simulink model "SurroundVehicleSensorFusion"  (R2022b)
settings: Solver=FixedStepAuto  StartTime=0.0  StopTime=scenario.StopTime  RelTol=1e-3  EnableMultiTasking=on
undefined symbols (not defined in the file): M, N, P, Q, trackAssignmentThreshold
libraries: motalgorithmslib x1, trackingutilitieslib x1
settings Model: Creator=The MathWorks, Inc.  LastModifiedBy=joelmiranda
settings SolverCC: AlgebraicLoopSolver=TrustRegion  MaxZcPerStep=1
settings DataIOCC: SaveOutput=off  SaveTime=off  ReturnWorkspaceOutputs=off
settings OptimizationCC: DefaultParameterBehavior=Inlined  InlineInvariantSignals=on  EnhancedBackFolding=on  PassReuseOutputArgsAs=Individual arguments  ZeroExternalMemoryAtStartup=off  ZeroInternalMemoryAtStartup=off  EfficientFloat2IntCast=on  OptimizeBlockOrder=speed  DifferentSizesBufferReuse=on  OptimizationCustomize=off  EfficientTunableParamExpr=on
settings DebuggingCC: ParameterPrecisionLossMsg=none  ParameterTunabilityLossMsg=error  UnconnectedInputMsg=warning  UnconnectedOutputMsg=warning  UnconnectedLineMsg=warning  ModelReferenceSymbolNameMessage=none  PregeneratedLibrarySubsystemCodeDiagnostic=none  SFMachineParentedDataDiag=warning  ArithmeticOperatorsInVariantConditions=warning
settings HardwareCC: ProdLongLongMode=on
settings ModelReferenceCC: EnableRefExpFcnMdlSchedulingChecks=on  PropagateVarSize=During execution
settings SFSimCC: SimUseLocalCustomCode=off  SimTargetLang=C++
settings RTWCC: Description=Embedded Coder  SystemTargetFile=ert.tlc  TemplateMakefile=ert_default_tmf  RTWVerbose=off  RTWUseLocalCustomCode=off  BuildConfiguration=Faster Runs  CodeExecutionProfiling=on  CodeProfilingSaveOptions=AllData  TargetLang=C++  DLArmComputeVersion=19.05
settings CodeAppCC: ForceParamTrailComments=on  IgnoreCustomStorageClasses=off  OperatorAnnotations=on  SimulinkDataObjDesc=on  SFDataObjDesc=on  CustomSymbolStrGlobalVar=$N$M  CustomSymbolStrType=$N$M_T  CustomSymbolStrFcn=APV_$N$M$F  CustomSymbolStrMacro=$N$M  InsertBlockDesc=on
settings ERTTargetCC: TargetLangStandard=C++03 (ISO)  GenerateSampleERTMain=on  CombineSignalStateStructs=on  CodeInterfacePackaging=C++ class  SupportVariableSizeSignals=on  InlinedParameterPlacement=NonHierarchical  RootIOFormat=Structure reference  ERTCustomFileTemplate=example_file_process.tlc
settings ConfigComp: CovScope=ReferencedModels  CovIncludeTopModel=off

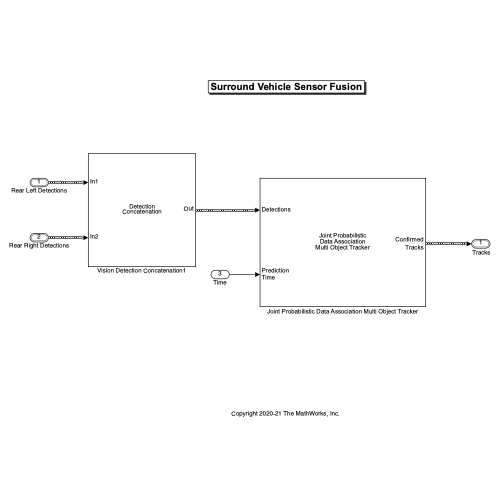
[thumbnail: Simulink's stored preview of the top-level diagram]
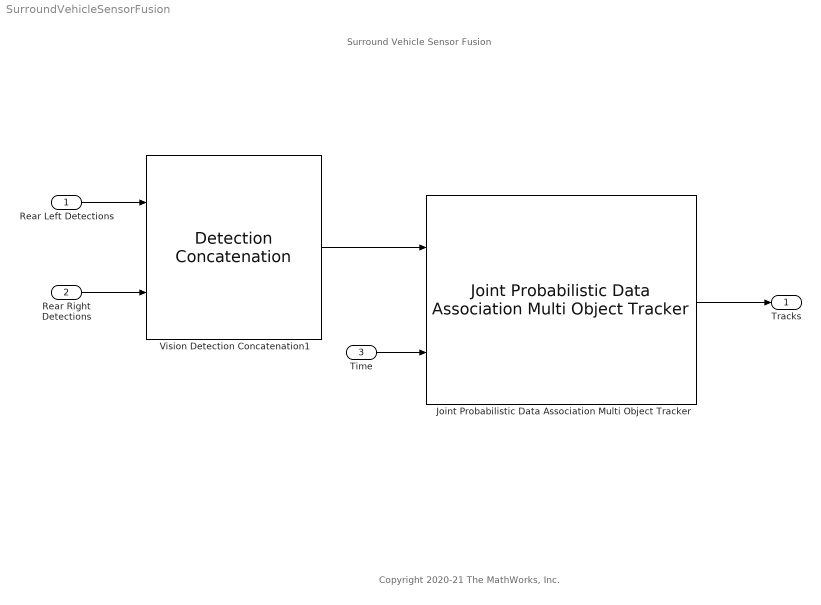
== system SurroundVehicleSensorFusion ==
  note: Surround Vehicle Sensor Fusion
  note: Copyright 2020-21 The MathWorks, Inc.
  Rear Left Detections : Inport  OutDataTypeStr=Bus: BusObjectDetections1  PortDimensions=[1 1]  SampleTime=[0.10000000000000001,0]  BusOutputAsStruct=on
  Rear Right Detections : Inport  Port=2  OutDataTypeStr=Bus: BusObjectDetections1  PortDimensions=[1 1]  SampleTime=[0.10000000000000001,0]  BusOutputAsStruct=on
  Time : Inport  Port=3  OutDataTypeStr=double  PortDimensions=[1 1]  SampleTime=[0.10000000000000001,0]
  Joint Probabilistic Data Association Multi Object Tracker : motalgorithmslib/Joint Probabilistic Data Association Multi Object Tracker  TrackerIndex=uint32( 0 )  FilterInitializationFcn=helperInitializeCVEKFFilter  MaxNumEvents=inf  EventGenerationFcn=jpdaEvents  MaxNumTracks=numTracks  MaxNumSensors=numSensors  TimeTolerance=1e-5  OOSMHandling=Terminate  MaxNumOOSMSteps=3  StateParametersSimulink=struct  HasStateParametersInput=off  EnableMemoryManagement=off  SimulateUsing=Interpreted execution  AssignmentThreshold=[ 1, Inf ] * trackAssignmentThreshold  InitializationThreshold=0  DetectionProbability=0.99  ClutterDensity=1e-7  TrackLogic=History  pHistoryConfThreshold=[ M, N ]  pHistoryDelThreshold=[ P, Q]  pIntegratedConfThreshold=0.95  pIntegratedDelThreshold=0.1  HitMissThreshold=trackRegisterThreshold  NewTargetDensity=1e-5  DeathRate=0.01  TimeInputSource=Input port  HasCostMatrixInput=off  HasDetectableTrackIDsInput=off  TentativeTracksOutputPort=off  AllTracksOutputPort=off  InfoOutputPort=off  BusNameSource=Property  BusName=BusTrackerJPDACameras  BusName2Source=Auto  BusName2=BusTrackerInfo  MaxNumDetectionsPerSensor=100  MaxNumDetectionsPerCluster=5  MaxNumTracksPerCluster=5  ClusterViolationHandling=Split and warn
  Vision Detection Concatenation1 : trackingutilitieslib/Detection Concatenation  NumInputs=2  BusNameSource=Auto  BusName=BusConcatenation  SimulateUsing=Interpreted execution
  " Tracks" : Outport  OutDataTypeStr=Bus: BusTrackerJPDACameras  BusOutputAsStruct=on
  wires:
  Time/1 -> Joint Probabilistic Data Association Multi Object Tracker/2
  Vision Detection Concatenation1/1 -> Joint Probabilistic Data Association Multi Object Tracker/1
  Rear Left Detections/1 -> Vision Detection Concatenation1/1
  Rear Right Detections/1 -> Vision Detection Concatenation1/2
  Joint Probabilistic Data Association Multi Object Tracker/1 -> " Tracks"/1
